simulink library "ModD_Controladores"  (R2018a)
settings: Solver=VariableStepAuto  StartTime=0.0  StopTime=10.0  RelTol=1e-3
undefined symbols (not defined in the file): PP_Controller
libraries: simulink x1
settings Model: Creator=Lisandro Cocca  LastModifiedBy=Lisandro Cocca

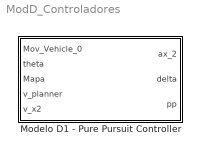
== system ModD_Controladores ==
  "Modelo D1 - Pure Pursuit Controller " : Subsystem  mask{kla=0, L=0, la_low=0, psi_max=0}
      mask prompts: kla "LA constant (kla)"; L "Axis separation (L)"; la_low "Ksoft (la_low)"; psi_max "Max SteerAng (rad)"

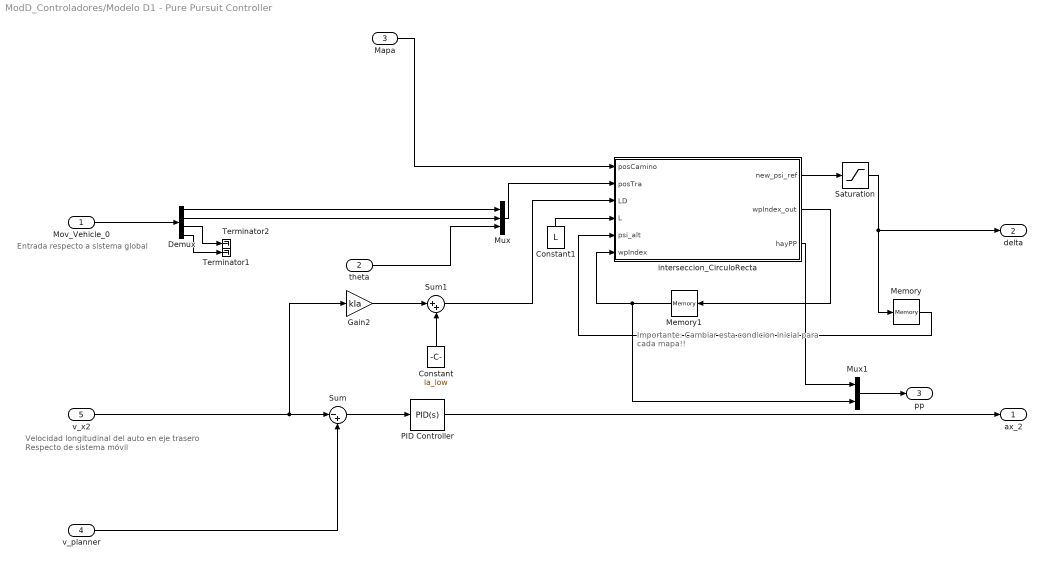
== system ModD_Controladores/Modelo D1 - Pure Pursuit Controller  ==
  note: Importante: Cambiar esta condicion inicial para cada mapa!!
  note: Entrada respecto a sistema global
  note: Velocidad longitudinal del auto en eje trasero
      | Respecto de sistema móvil
  Mov_Vehicle_0 : Inport
  theta : Inport  Port=2
  Mapa : Inport  Port=3
  v_planner : Inport  Port=4
  v_x2 : Inport  Port=5
  Constant : Constant  Value=la_low  VectorParams1D=off
  Constant1 : Constant  Value=L
  Demux : Demux
  Gain2 : Gain  Gain=kla
  Memory : Memory  InheritSampleTime=on  LinearizeMemory=on  LinearizeAsDelay=on
  Memory1 : Memory  InheritSampleTime=on  LinearizeMemory=on  LinearizeAsDelay=on
  Mux : Mux  Inputs=3
  Mux1 : Mux  Inputs=2
  PID Controller : simulink/Continuous/PID Controller  Controller=PID  TimeDomain=Continuous-time  SampleTime=-1  IntegratorMethod=Forward Euler  FilterMethod=Forward Euler  Form=Parallel  UseFilter=on  ControllerParametersSource=internal  P=PP_Controller.KP  I=PP_Controller.KI  D=PP_Controller.KD  N=100  InitialConditionSource=internal  InitialConditionForIntegrator=0  InitialConditionForFilter=0  ExternalReset=none  LimitOutput=on  UpperSaturationLimit=inf  LowerSaturationLimit=-inf  LinearizeAsGain=on  AntiWindupMode=none  Kb=1  TrackingMode=off  Kt=1  PParamMin=[]  PParamMax=[]  IParamMin=[]  IParamMax=[]  DParamMin=[]  DParamMax=[]  NParamMin=[]  NParamMax=[]  KbParamMin=[]  KbParamMax=[]  KtParamMin=[]  KtParamMax=[]  POutMin=[]  POutMax=[]  IOutMin=[]  IOutMax=[]  DOutMin=[]  DOutMax=[]  NOutMin=[]  NOutMax=[]  KbOutMin=[]  KbOutMax=[]  KtOutMin=[]  KtOutMax=[]  IntegratorOutMin=[]  IntegratorOutMax=[]  FilterOutMin=[]  FilterOutMax=[]  SumOutMin=[]  SumOutMax=[]  SumI1OutMin=[]  SumI1OutMax=[]  SumI2OutMin=[]  SumI2OutMax=[]  SumI3OutMin=[]  SumI3OutMax=[]  SumDOutMin=[]  SumDOutMax=[]  SaturationOutMin=[]  SaturationOutMax=[]  IntegratorContinuousStateAttributes=''  IntegratorStateMustResolveToSignalObject=off  IntegratorRTWStateStorageClass=Auto  FilterContinuousStateAttributes=''  FilterStateMustResolveToSignalObject=off  FilterRTWStateStorageClass=Auto  DifferentiatorICPrevScaledInput=0  DifferentiatorOutMin=[]  DifferentiatorOutMax=[]  FilterDiffOutCoefMin=[]  FilterDiffOutCoefMax=[]  SumDenOutMin=[]  SumDenOutMax=[]  SumNumOutMin=[]  SumNumOutMax=[]  ReciprocalOutMin=[]  ReciprocalOutMax=[]  DivideOutMin=[]  DivideOutMax=[]  TunerSelectOption=Transfer Function Based (PID Tuner App)
  Saturation : Saturate  UpperLimit=psi_max  LowerLimit=-psi_max  LinearizeAsGain=off
  Sum : Sum  Inputs=|-+
  Sum1 : Sum  Inputs=|++
  Terminator1 : Terminator
  Terminator2 : Terminator
  interseccion_CirculoRecta : MATLAB Function  TreatAsAtomicUnit=on
  ax_2 : Outport
  delta : Outport  Port=2
  pp : Outport  Port=3
  wires:
  Mov_Vehicle_0/1 -> Demux/1
  theta/1 -> Mux/3
  Demux/2 -> Mux/2
  Mux/1 -> interseccion_CirculoRecta/2(posTra)
  Demux/4 -> Terminator1/1
  Sum/1 -> PID Controller/1
  PID Controller/1 -> ax_2/1
  Demux/1 -> Mux/1
  Sum1/1 -> interseccion_CirculoRecta/3(LD)
  Gain2/1 -> Sum1/1
  Constant/1 -> Sum1/2
  Constant1/1 -> interseccion_CirculoRecta/4(L)
  Memory/1 -> interseccion_CirculoRecta/5(psi_alt)
  interseccion_CirculoRecta/1(new_psi_ref) -> Saturation/1
  Saturation/1 -> delta/1, Memory/1
  Mapa/1 -> interseccion_CirculoRecta/1(posCamino)
  interseccion_CirculoRecta/2(wpIndex_out) -> Memory1/1
  Memory1/1 -> Mux1/2, interseccion_CirculoRecta/6(wpIndex)
  v_planner/1 -> Sum/2
  v_x2/1 -> Sum/1, Gain2/1
  Demux/3 -> Terminator2/1
  interseccion_CirculoRecta/3(hayPP) -> Mux1/1
  Mux1/1 -> pp/1

== matlab function ModD_Controladores/Modelo D1 - Pure Pursuit Controller /interseccion_CirculoRecta ==
  data: new_psi_ref output; posCamino input; posTra input; LD input; L input; psi_alt input; wpIndex input; wpIndex_out output; hayPP output
function [new_psi_ref, wpIndex_out, hayPP]= interseccion_CirculoRecta(posCamino, posTra, LD, L, psi_alt, wpIndex)

wpSize = 1000; % CANTIDAD DE WAYPOINTS USADOS PARA EVALUAR LA INTERSECCION
wpIndex_max = wpIndex + wpSize/2;
wpIndex_min = wpIndex - wpSize/2;

% Si esta min o max estan fuera de los límites, agrego el sobrante en el
% otro extremo
if wpIndex_min < 1
    wpIndex_max = wpIndex_max + wpIndex - wpIndex_min;
    wpIndex_min = 1;
end
if wpIndex_max > length(posCamino)
    wpIndex_min = wpIndex_min + wpIndex - wpIndex_max;
    wpIndex_max = length(posCamino);
end

% Filtro el camino
posCamino_filtrado = posCamino([wpIndex_min:wpIndex_max]',:);

posTrasero = transpose(posTra);
intersecciones = [];
for i = 1:length(posCamino_filtrado)-1
    deltaR = posCamino_filtrado(i+1,1:2) - posCamino_filtrado(i,1:2);
    deltaC = posCamino_filtrado(i,1:2)- posTrasero(1:2);
    a = deltaR(1)^2 + deltaR(2)^2;
    b = 2*(deltaR(1)*deltaC(1) + deltaR(2)*deltaC(2));
    c = deltaC(1)^2 + deltaC(2)^2 - LD ^2;
    u_aux = roots([a,b,c]);
    if imag(u_aux) == 0
        u = real(u_aux);
    else
        u = [];
    end
    for j = 1:length(u)
        if u(j)>=0 && u(j)<1
            aux = [posCamino_filtrado(i,1) + deltaR(1)*u(j), posCamino_filtrado(i,2) + deltaR(2)*u(j), i+u(j)];
            intersecciones = [intersecciones ; aux];
        end
    end
end

if isempty(intersecciones)
    new_psi_ref = psi_alt;
    wpIndex_out = wpIndex;
    hayPP = 0;
else
    indexGlobal = round(max(intersecciones(:,3))); % El elemento 3 es el valor del indice
    [~, index] = max(intersecciones(:,3)); % El elemento 3 es el valor del indice
    intFinal = intersecciones(index,:); % Es la interseccion mas avanzada en el camino
    
    error_global = transpose(intFinal(1:2) - posTrasero(1:2)); % Vector Error en sistema global
    
    a11 = cos(posTrasero(3));
    a12 = sin(posTrasero(3));
    a21 = -sin(posTrasero(3));
    a22 = cos(posTrasero(3));
    A = [[a11,a12];[a21,a22]];
    
    error_loc = A*error_global;
   
    new_psi_ref = atan(2 * L * error_loc(2) / (LD^2));
    wpIndex_out = indexGlobal + wpIndex_min - 1;
    hayPP = 1;
end
end
